simulink model "dyskretyzacja1_granica_stablinosci"  (R2018b)
settings: Solver=FixedStepDiscrete  StartTime=0.0  StopTime=10  FixedStep=T  RelTol=1e-3
values from neighbouring files (symbols this model uses):
  T = 1    [nyquist.m]    (also in oscylacje_reczne.m)
settings Model: Creator=Dominik  LastModifiedBy=user
settings DebuggingCC: LibraryContextMissingDiagnostic=none
settings SFSimCC: SimUseLocalCustomCode=off
settings RTWCC: RTWUseLocalCustomCode=off

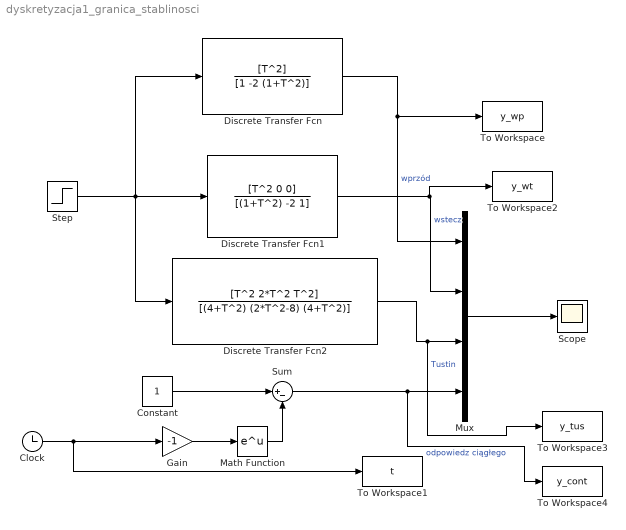
== system dyskretyzacja1_granica_stablinosci ==
  Clock : Clock
  Constant : Constant
  Discrete Transfer Fcn : DiscreteTransferFcn  Numerator=[T^2]  Denominator=[1 -2 (1+T^2)]  SampleTime=T
  Discrete Transfer Fcn1 : DiscreteTransferFcn  Numerator=[T^2 0 0]  Denominator=[(1+T^2) -2 1]  SampleTime=T
  Discrete Transfer Fcn2 : DiscreteTransferFcn  Numerator=[T^2 2*T^2 T^2]  Denominator=[(4+T^2) (2*T^2-8) (4+T^2)]  SampleTime=T
  Gain : Gain  Gain=-1
  Math Function : Math  SaturateOnIntegerOverflow=on
  Mux : Mux
  Scope : Scope
  Step : Step  Time=0  SampleTime=0
  Sum : Sum  Inputs=|+-
  To Workspace : ToWorkspace  VariableName=y_wp  SampleTime=-1
  To Workspace1 : ToWorkspace  VariableName=t  SampleTime=-1
  To Workspace2 : ToWorkspace  VariableName=y_wt  SampleTime=-1
  To Workspace3 : ToWorkspace  VariableName=y_tus  SampleTime=-1
  To Workspace4 : ToWorkspace  VariableName=y_cont  SampleTime=-1
  wires:
  Gain/1 -> Math Function/1
  Clock/1 -> To Workspace1/1, Gain/1
  Constant/1 -> Sum/1
  Math Function/1 -> Sum/2
  Sum/1 -> To Workspace4/1, Mux/4  "odpowiedz ciągłego"
  Discrete Transfer Fcn/1 -> To Workspace/1, Mux/1  "wprzód"
  Discrete Transfer Fcn2/1 -> To Workspace3/1, Mux/3  "Tustin"
  Discrete Transfer Fcn1/1 -> To Workspace2/1, Mux/2  "wstecz"
  Mux/1 -> Scope/1
  Step/1 -> Discrete Transfer Fcn1/1, Discrete Transfer Fcn2/1, Discrete Transfer Fcn/1
